simulink subsystem "FF_reconstructor"  (R2024b)
settings: Solver=VariableStepAuto  StartTime=0.0  StopTime=10.0  RelTol=1e-3
undefined symbols (not defined in the file or in its folder): References
settings Model: Creator=thesa  LastModifiedBy=jack
settings RTWCC: GPUComputeCapability=3.5

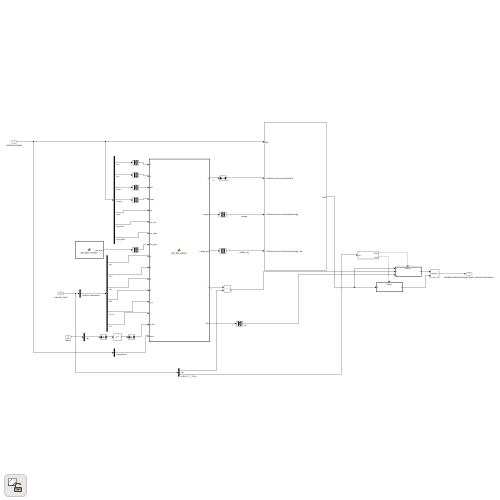
[thumbnail: Simulink's stored preview of the top-level diagram]
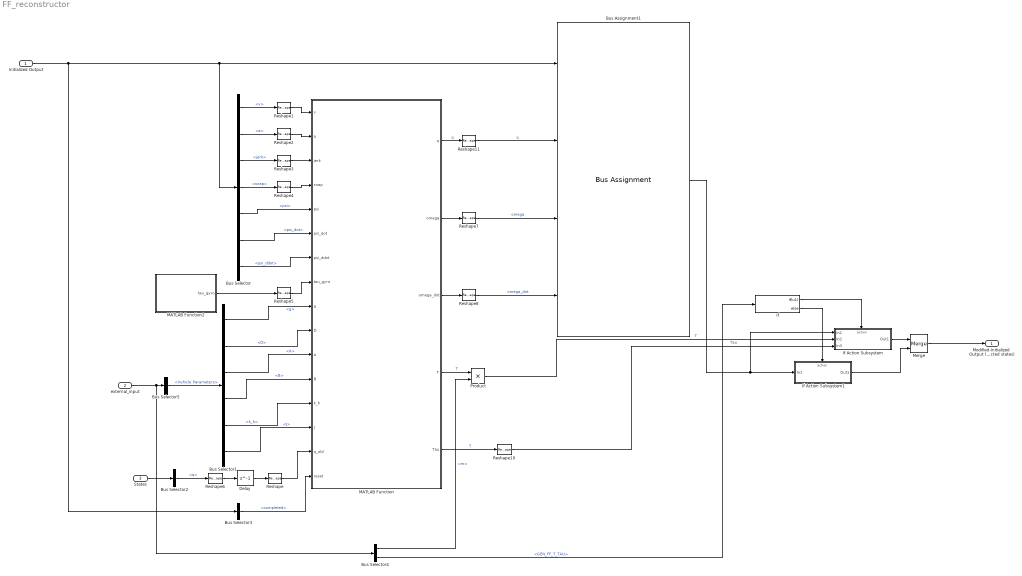
== system FF_reconstructor ==
  Initialized Output : Inport
  external_input : Inport  Port=2
  States : Inport  Port=3
  Bus Assignment1 : BusAssignment  AssignedSignals=References.reconstructed.q,References.reconstructed.omega,References.reconstructed.omega_dot
  Bus Selector : BusSelector  OutputSignals=References.trajectory.v,References.trajectory.a,References.trajectory.jerk,References.trajectory.snap,References.trajectory.psi,References.trajectory.psi_dot,References.trajectory.psi_ddot
  Bus Selector1 : BusSelector  OutputSignals=g,D,A,B,k_h,J
  Bus Selector2 : BusSelector  OutputSignals=q
  Bus Selector3 : BusSelector  OutputSignals=References.completed
  Bus Selector4 : BusSelector  OutputSignals=Vehicle Parameters.m,Pilot Input.Parameters.GEN_FF_T_TAU
  Bus Selector5 : BusSelector  OutputSignals=Vehicle Parameters
  Delay : Delay  DelayLength=1  InitialCondition=[1,0,0,0]
  If : If  IfExpression=u1
  If Action Subsystem : Subsystem  TreatAsAtomicUnit=on
  If Action Subsystem1 : Subsystem  TreatAsAtomicUnit=on
  MATLAB Function : MATLAB Function  TreatAsAtomicUnit=on
  MATLAB Function2 : MATLAB Function  TreatAsAtomicUnit=on
  Merge : Merge
  Product : Product
  Reshape : Reshape  OutputDimensionality=Row vector (2-D)
  Reshape{1..5,7..8,10} (8 alike) : Reshape  OutputDimensionality=Column vector (2-D)
  Reshape11 : Reshape  OutputDimensionality=Row vector (2-D)
  Reshape6 : Reshape  OutputDimensionality=Row vector (2-D)
  Modified-Initialized Output (with reconstructed states) : Outport
  wires:
  Bus Selector3/1 -> MATLAB Function/16(reset)  "<completed>"
  Reshape11/1 -> Bus Assignment1/2  "q"
  Reshape8/1 -> Bus Assignment1/4  "omega_dot"
  Reshape7/1 -> Bus Assignment1/3  "omega"
  Reshape6/1 -> Delay/1
  Reshape/1 -> MATLAB Function/15(q_old)
  Reshape5/1 -> MATLAB Function/8(tau_gyro)
  Reshape4/1 -> MATLAB Function/4(snap)
  Reshape3/1 -> MATLAB Function/3(jerk)
  Reshape2/1 -> MATLAB Function/2(a)
  Reshape1/1 -> MATLAB Function/1(v)
  MATLAB Function/3(omega_dot) -> Reshape8/1
  MATLAB Function/1(q) -> Reshape11/1  "q"
  MATLAB Function/2(omega) -> Reshape7/1
  MATLAB Function2/1(tau_gyro) -> Reshape5/1
  Delay/1 -> Reshape/1
  Bus Selector2/1 -> Reshape6/1  "<q>"
  States/1 -> Bus Selector2/1
  Bus Selector1/6 -> MATLAB Function/14(J)  "<J>"
  Bus Selector1/5 -> MATLAB Function/13(k_h)  "<k_h>"
  Bus Selector1/4 -> MATLAB Function/12(B)  "<B>"
  Bus Selector1/3 -> MATLAB Function/11(A)  "<A>"
  Bus Selector1/2 -> MATLAB Function/10(D)  "<D>"
  Bus Selector1/1 -> MATLAB Function/9(g)  "<g>"
  Bus Selector5/1 -> Bus Selector1/1  "<Vehicle Parameters>"
  Bus Selector/7 -> MATLAB Function/7(psi_ddot)  "<psi_ddot>"
  Bus Selector/6 -> MATLAB Function/6(psi_dot)  "<psi_dot>"
  Bus Selector/5 -> MATLAB Function/5(psi)  "<psi>"
  Bus Selector/4 -> Reshape4/1  "<snap>"
  Bus Selector/3 -> Reshape3/1  "<jerk>"
  Bus Selector/2 -> Reshape2/1  "<a>"
  Bus Selector/1 -> Reshape1/1  "<v>"
  Initialized Output/1 -> Bus Selector3/1, Bus Assignment1/1, Bus Selector/1
  MATLAB Function/4(T) -> Product/1  "T"
  Bus Selector4/1 -> Product/2  "<m>"
  Reshape10/1 -> If Action Subsystem/3(In3)  "Tau"
  Product/1 -> If Action Subsystem/2(In2)  "T"
  external_input/1 -> Bus Selector5/1, Bus Selector4/1
  Bus Selector4/2 -> If/1  "<GEN_FF_T_TAU>"
  MATLAB Function/5(Tau) -> Reshape10/1  "T"
  If/1 -> If Action Subsystem/Action
  If/2 -> If Action Subsystem1/Action
  Bus Assignment1/1 -> If Action Subsystem1/1(In1), If Action Subsystem/1(In1)
  If Action Subsystem/1(Out1) -> Merge/1
  If Action Subsystem1/1(Out1) -> Merge/2
  Merge/1 -> Modified-Initialized Output (with reconstructed states)/1

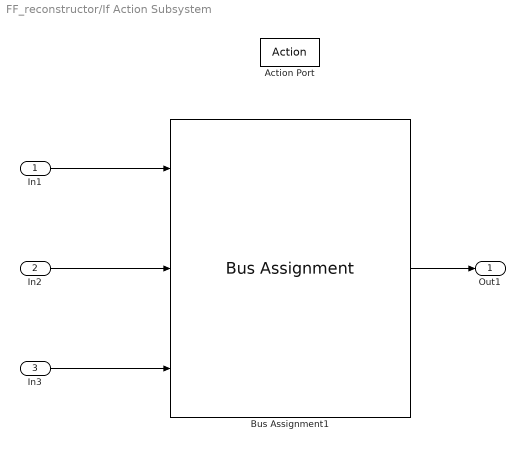
== system FF_reconstructor/If Action Subsystem ==
  In1 : Inport
  In2 : Inport  Port=2
  In3 : Inport  Port=3
  Action Port : ActionPort
  Bus Assignment1 : BusAssignment  AssignedSignals=References.reconstructed.T,References.reconstructed.Tau
  Out1 : Outport
  wires:
  In3/1 -> Bus Assignment1/3
  In2/1 -> Bus Assignment1/2
  Bus Assignment1/1 -> Out1/1
  In1/1 -> Bus Assignment1/1

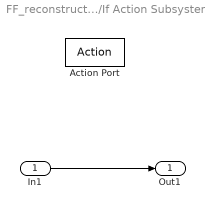
== system FF_reconstructor/If Action Subsystem1 ==
  In1 : Inport
  Action Port : ActionPort
  Out1 : Outport
  wires:
  In1/1 -> Out1/1

== matlab function FF_reconstructor/MATLAB Function ==
  data: v input; q output size=[1 ,4]; a input; jerk input; snap input; psi input; psi_dot input; psi_ddot input; tau_gyro input; g input; D input; A input; B input; k_h input; J input; q_old input; omega output; omega_dot output; T output; Tau output; reset input
function [q, omega, omega_dot, T, Tau] = ...
    get_flat_states(...
    v, a, jerk, snap, psi, psi_dot, psi_ddot,...
    tau_gyro,...
    g, D, A, B, k_h, J, ...
    q_old, reset)

[q, omega, omega_dot, T, Tau] = ...
    get_flat_states(...
    v, a, jerk, snap, psi, psi_dot, psi_ddot,...
    tau_gyro,...
    g, D, A, B, k_h, J, ...
    q_old, reset);
end

== matlab function FF_reconstructor/MATLAB Function2 ==
  data: tau_gyro output
function tau_gyro = get_gyro_torque
tau_gyro = get_gyro_torque;
end
